simulink model "Metal_detector_model_test"  (R2022b)
settings: Solver=VariableStepAuto  StartTime=0.0  StopTime=7e-3  MaxStep=1/300e3  RelTol=1e-3  AbsTol=1e-3
model workspace (MAT data in the model file):
  airGap = 1
libraries: fl_lib x6, nesl_utility x3, ee_lib x2
settings Model: Creator=chrislee  LastModifiedBy=ASUS
settings SolverCC: AutoScaleAbsTol=off  AlgebraicLoopSolver=TrustRegion  MaxZcPerStep=1
settings DebuggingCC: UnconnectedInputMsg=warning  UnconnectedOutputMsg=warning  UnconnectedLineMsg=warning  SymbolicDimsDataTypeCodeGenerationDiagnostic=none  SFMachineParentedDataDiag=warning
settings ModelReferenceCC: EnableRefExpFcnMdlSchedulingChecks=on
settings SFSimCC: CustomCodeUndefinedFunction=UseInterfaceOnly
settings RTWCC: DLArmComputeVersion=19.05
settings SimscapeCC: SimscapeLogType=all  SimscapeLogSimulationStatistics=on  SimscapeLogDataHistory=10000

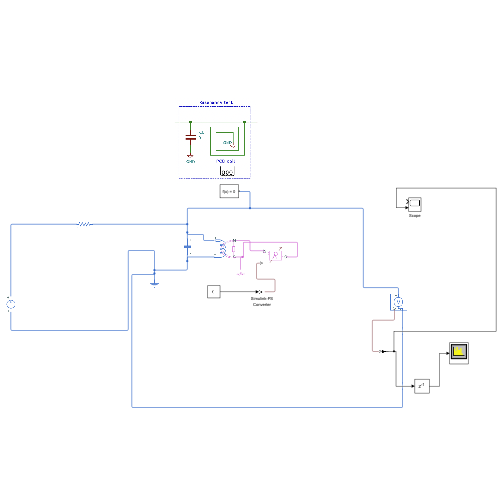
[thumbnail: Simulink's stored preview of the top-level diagram]
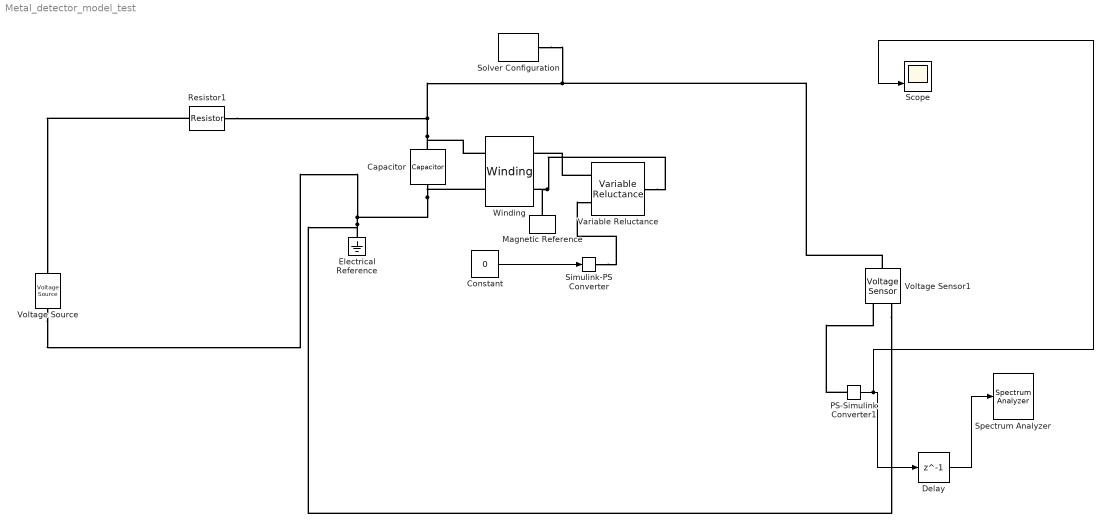
== system Metal_detector_model_test ==
  Capacitor : fl_lib/Electrical/Electrical Elements/Capacitor  c=47 nF  r=1e-6 Ohm  g=0 1/Ohm  i_specify=off  i_priority=None  i=0 A  i_nominal_specify=off  i_nominal_unit=A  i_nominal_value=1  v_specify=off  v_priority=None  v=0 V  v_nominal_specify=off  v_nominal_unit=V  v_nominal_value=1  vc_specify=off  vc_priority=High  vc=0 V  vc_nominal_specify=off  vc_nominal_unit=V  vc_nominal_value=1
  Constant : Constant  Value=0
  Delay : Delay  DelayLength=1  InitialCondition=0
  Electrical Reference : fl_lib/Electrical/Electrical Elements/Electrical Reference
  Magnetic Reference : fl_lib/Magnetic/Magnetic Elements/Magnetic Reference
      settings: InternalSimscapePortConfiguration="{\"Bottom\":[],\"Left\":[{\"id\":\"M\",\"label\":\"\",\"type\":\"foundation.magnetic.magnetic\"}],\"Right\":[],\"Top\":[]}"
  PS-Simulink Converter1 : nesl_utility/PS-Simulink Converter  PhysicalDomain=network_engine_domain  SubClassName=ps_output  LeftPortType=input  RightPortType=output  PseudoPeriodic=off  Frequencies=[]  VectorFormat=inherit  Unit=inherit  AffineConversion=off
  Resistor1 : fl_lib/Electrical/Electrical Elements/Resistor  R=100 Ohm  i_specify=off  i_priority=None  i=0 A  i_nominal_specify=off  i_nominal_unit=A  i_nominal_value=1  v_specify=off  v_priority=None  v=0 V  v_nominal_specify=off  v_nominal_unit=V  v_nominal_value=1
  Scope : Scope  NumInputPorts=2
  Simulink-PS Converter : nesl_utility/Simulink-PS Converter  PhysicalDomain=network_engine_domain  SubClassName=ps_input  LeftPortType=input  RightPortType=output  PseudoPeriodic=off  Frequencies=[]  NoiseDistribution=none  NoiseParameters=[]  Unit=1  AffineConversion=off  FilteringAndDerivatives=provide  SimscapeFilterOrder=1  InputFilterTimeConstant=0.001  UdotUserProvided=0
  Solver Configuration : nesl_utility/Solver Configuration  PhysicalDomain=network_engine_domain  SubClassName=solver  LeftPortType=input  RightPortType=generic  Tones=[]  Harmonics=[]  SimulateNoise=off  Profile=off  UseLocalSampling=off  EnableSwitchedLinearOptims=on  FrequencyDomain=off  UseCCode=off  RelTol=0.001  AbsTol=0.001  MinStep=1e-09  ToWorkspace=off  RevertToSquareIcSolve=off  NumHomotopyIterations=100  PhasorMode=off  PhasorModeNumHarmonics=1  ConsistencySolver=NEWTON_FTOL  IndexReductionMethod=DerivativeReplacement  DoDC=off  ResidualTolerance=1e-09  ConsistencyTolSource=GLOBAL  ConsistencyAbsTol=0.001  ConsistencyRelTol=0.001  ConsistencyTolFactor=0.001  UseLocalSolver=off  LocalSolverChoice=NE_BACKWARD_EULER_ADVANCER  ResolveIndetEquations=on  FunctionEvalNumThread=1  LocalSolverSampleTime=0.001  DoFixedCost=off  MaxNonlinIter=3  MaxModeIter=2  ComputeImpulses=off  ImpulseIterations=2  LinearAlgebra=auto  LinearAlgebraNumThread=0  EquationFormulation=NE_TIME_EF  DelaysMemoryBudget=1024  AutomaticFiltering=on  FilteringTimeConstant=0.001  PartitionStorageMethod=AS_NEEDED  PartitionMemoryBudget=1024  PartitionMethod=ROBUST
  Spectrum Analyzer : SpectrumAnalyzer
  Variable Reluctance : fl_lib/Magnetic/Magnetic Elements/Variable Reluctance  Xmin=0 m  CSA=0.01 m^2  mur=10  phi_specify=off  phi_priority=None  phi=0 Wb  phi_nominal_specify=off  phi_nominal_unit=Wb  phi_nominal_value=1  mmf_specify=off  mmf_priority=None  mmf=0 A  mmf_nominal_specify=off  mmf_nominal_unit=A  mmf_nominal_value=1
      settings: InternalSimscapePortConfiguration="{\"Bottom\":[],\"Left\":[{\"id\":\"N\",\"label\":\"N\",\"type\":\"foundation.magnetic.magnetic\"},{\"id\":\"X\",\"label\":\"\",\"type\":\"input\"}],\"Right\":[{\"id\":\"S\",\"label\":\"S\",\"type\":\"foundation.magnetic.magnetic\"}],\"Top\":[]}"
  Voltage Sensor1 : fl_lib/Electrical/Electrical Sensors/Voltage Sensor
  Voltage Source : ee_lib/Sources/Voltage Source  dc_voltage=0 V  ac_voltage=0 V  ac_shift=0 rad  ac_frequency=60 Hz  noise_mode=1  PSD=1 V^2/Hz  sample_time=1/500e3 s  repeatability=1  user_seed=0  auto_seed=3499211588  i_specify=off  i_priority=None  i=0 A  i_nominal_specify=off  i_nominal_unit=A  i_nominal_value=1  v_specify=off  v_priority=None  v=0 V  v_nominal_specify=off  v_nominal_unit=V  v_nominal_value=1
  Winding : ee_lib/Passive/Winding  Nw=10  Rw=1e-3 Ohm  Rl=1e5 1/H  Gw=0 1/Ohm  thermalPort=simscape.enum.thermaleffects.omit  alpha=3.93e-3 1/K  Tmeas=25 degC  winding_thermal_mass=100 J/K  enable_faults=simscape.enum.onoff.off  lambdaPercent=50  fault_action=simscape.enum.assert.action.none  turnsShort=ee.enum.faults.faultTurnsShort.no  openCct=ee.enum.faults.faultTurnsOpenCkt.no  groundShort=ee.enum.faults.faultTurnsGroundShort.no  groundShortG=0 1/Ohm  tau_fault=1e-3 s  enable_temporal_fault=ee.enum.faults.faultTriggerTemporal.no  t_fault=1 s  enable_behavioral_fault=ee.enum.faults.faultTriggerBehavioral.no  max_permissible_voltage=100 V  n_fail_on_voltage=1  max_permissible_current=1 A  t_fail_on_current=1 s  T_specify=off  T_priority=None  T=25 degC  T_nominal_specify=off  T_nominal_unit=degC  T_nominal_value=1  i_specify=off  i_priority=None  i=0 A  i_nominal_specify=off  i_nominal_unit=A  i_nominal_value=1  v_specify=off  v_priority=None  v=0 V  v_nominal_specify=off  v_nominal_unit=V  v_nominal_value=1  phi_specify=off  phi_priority=None  phi=0 Wb  phi_nominal_specify=off  phi_nominal_unit=Wb  phi_nominal_value=1  power_dissipated_specify=off  power_dissipated_priority=None  power_dissipated=0 W  power_dissipated_nominal_specify=off  power_dissipated_nominal_unit=W  power_dissipated_nominal_value=1
      settings: InternalSimscapePortConfiguration="{\"Bottom\":[],\"Left\":[{\"id\":\"p\",\"label\":\"+\",\"type\":\"foundation.electrical.electrical\"},{\"id\":\"n\",\"label\":\"-\",\"type\":\"foundation.electrical.electrical\"}],\"Right\":[{\"id\":\"N\",\"label\":\"N\",\"type\":\"foundation.magnetic.magnetic\"},{\"id\":\"S\",\"label\":\"S\",\"type\":\"foundation.magnetic.magnetic\"}],\"Top\":[]}"
  wires:
  PS-Simulink Converter1/1 -> Scope/2, Delay/1
  Delay/1 -> Spectrum Analyzer/1
  Constant/1 -> Simulink-PS Converter/1
  connections:
  Capacitor/RConn1 -- Voltage Source/RConn1 -- Voltage Sensor1/RConn2 -- Electrical Reference/LConn1 -- Winding/LConn2
  PS-Simulink Converter1/LConn1 -- Voltage Sensor1/RConn1
  Capacitor/LConn1 -- Voltage Sensor1/LConn1 -- Solver Configuration/RConn1 -- Resistor1/LConn1 -- Winding/LConn1
  Resistor1/RConn1 -- Voltage Source/LConn1
  Variable Reluctance/LConn1 -- Winding/RConn1
  Variable Reluctance/RConn1 -- Magnetic Reference/LConn1 -- Winding/RConn2
  Simulink-PS Converter/RConn1 -- Variable Reluctance/LConn2
